simulink model "test"  (R2018b)
settings: Solver=VariableStepAuto  StartTime=0.0  StopTime=100  MaxStep=0.01  RelTol=1e-3
settings Model: Creator=kekos  LastModifiedBy=kekos

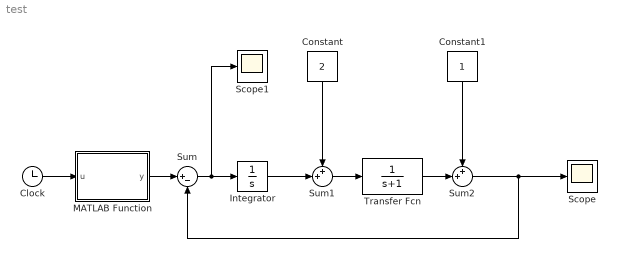
== system test ==
  Clock : Clock
  Constant : Constant  Value=2
  Constant1 : Constant
  Integrator : Integrator
  MATLAB Function : MATLAB Function  TreatAsAtomicUnit=on
  Scope : Scope
  Scope1 : Scope
  Sum : Sum  Inputs=|+-
  Sum1 : Sum  Inputs=++|
  Sum2 : Sum  Inputs=++|
  Transfer Fcn : TransferFcn  Denominator=[1 1]
  wires:
  Clock/1 -> MATLAB Function/1(u)
  MATLAB Function/1(y) -> Sum/1
  Constant1/1 -> Sum2/1
  Constant/1 -> Sum1/1
  Sum1/1 -> Transfer Fcn/1
  Transfer Fcn/1 -> Sum2/2
  Integrator/1 -> Sum1/2
  Sum/1 -> Scope1/1, Integrator/1
  Sum2/1 -> Scope/1, Sum/2

== matlab function test/MATLAB Function ==
  data: u input; y output
function y = fcn(u)

y = 2*u;
